simulink model "stwart_platform_model"  (R2026a)
settings: Solver=VariableStepAuto
undefined symbols (not defined in the file): X, Y, Z
libraries: sm_lib x64, nesl_utility x7
(part 3 of 3)

== matlab function stwart_platform_model/MATLAB Function ==
  data: x input; out1 output; out2 output; out3 output; out4 output; out5 output; data output; out6 output; y input; z input; roll input; pitch input; yaw input
function [out1, out2, out3, out4, out5, data, out6] = fcn(x, y, z, roll, pitch, yaw)
% Geometry inputs
outer_base_dia = 260;
inner_base_dia = 200;
R_base = (outer_base_dia + inner_base_dia) / 4; % Radius = 115 mm

outer_plat_dia = 160;
inner_plat_dia = 100;
R_plat = (outer_plat_dia + inner_plat_dia) / 4; % Radius = 65 mm

% Angular spacing for joint pairs (in degrees)
beta_base = 15;  % Half-angle separation for base joint pairs
beta_plat = 10;  % Half-angle separation for platform joint pairs

base_angles_deg = [60 - beta_base,  60 + beta_base, ...
    180 - beta_base, 180 + beta_base, ...
    300 - beta_base, 300 + beta_base];

plat_angles_deg = [60 - beta_plat,  60 + beta_plat, ...
    180 - beta_plat, 180 + beta_plat, ...
    300 - beta_plat, 300 + beta_plat];

% Convert angles to radians
base_angles = deg2rad(base_angles_deg);
plat_angles = deg2rad(plat_angles_deg);

% Base joint vectors B_i in Base Frame (3x6 matrix)
B = [R_base * cos(base_angles);
    R_base * sin(base_angles);
    zeros(1, 6)];

% Platform joint vectors P_i in Platform Frame (3x6 matrix)
P = [R_plat * cos(plat_angles);
    R_plat * sin(plat_angles);
    zeros(1, 6)];

% Translation vector from dynamic inputs
T = [x; y; z]; 

% Target orientation angles (convert degrees to radians)
phi   = deg2rad(roll);   % Roll (X-axis rotation)
theta = deg2rad(pitch);  % Pitch (Y-axis rotation)
psi   = deg2rad(yaw);    % Yaw (Z-axis rotation)

% Rotation matrices
Rx = [1, 0, 0; 
    0, cos(phi), -sin(phi); 
    0, sin(phi), cos(phi)];

Ry = [cos(theta), 0, sin(theta); 
    0, 1, 0; 
    -sin(theta), 0, cos(theta)];

Rz = [cos(psi), -sin(psi), 0; 
    sin(psi), cos(psi), 0; 
    0, 0, 1];

R = Rz * Ry * Rx; % Combined rotation matrix (ZYX order)

leg_lengths = zeros(1, 6);

for i = 1:6
    % Transform platform joint i to base frame: p_i = T + R * P_i
    p_i = T + R * P(:, i);

    % Vector along the prismatic leg: S_i = p_i - B_i
    S_i = p_i - B(:, i);

    % Leg length L_i = norm(S_i)
    leg_lengths(i) = norm(S_i);
end

% Assign each output explicitly
out1 = leg_lengths(1);
out2 = leg_lengths(2);
out3 = leg_lengths(3);
out4 = leg_lengths(4);
out5 = leg_lengths(5);
out6 = leg_lengths(6);
end
